simulink model "mmc"  (R2023b)
settings: Solver=VariableStepAuto  StartTime=0.0  StopTime=2  RelTol=1e-3
values from neighbouring files (symbols this model uses):
  ab0_to_cell = inv(cell_to_2ab0)    [init_mmc.m]
  cell_to_2ab0 = kron(abc_to_ab0, abc_to_ab0)    [init_mmc.m]
  grid_to_cell = kron(eye(3), ones(3, 1))    [init_mmc.m]
  J = [0 -1; 1 0]    [SafetyFilterSystemDPC.m]    (also in init_mmc.m)
  machine_to_cell = kron(ones(3, 1), eye(3))    [init_mmc.m]
  volt_to_cell = [      [          1 0 0 0 0 0 ... (first row only)    [init_mmc.m]
undefined symbols (not defined in the file or in its folder): cpu, ctrl, DiscIntNeverNeededParam, fdesignblkfcn, gcbh, grid, load1, machine, mmc, pq_ctrl, sim, soa
libraries: eeDiscretePi x9, spsabctodq0Lib x9, spsThreePhaseSeriesRLCBranchLib x8, dsparch4 x6, spsControlledVoltageSourceLib x6, spsThreePhaseVIMeasurementLib x6, eeGeneralControl x5, spsBreakerLib x3, spsGroundLib x3, library x3, spsThreePhaseBreakerLib x2, spsdq0toabcLib x2
(part 1 of 2)
settings Model: SimulationMode=accelerator  Creator=ma1155716  LastModifiedBy=ma1155716

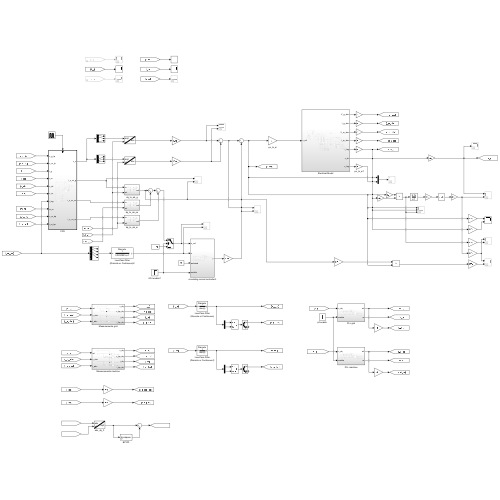
[thumbnail: Simulink's stored preview of the top-level diagram]
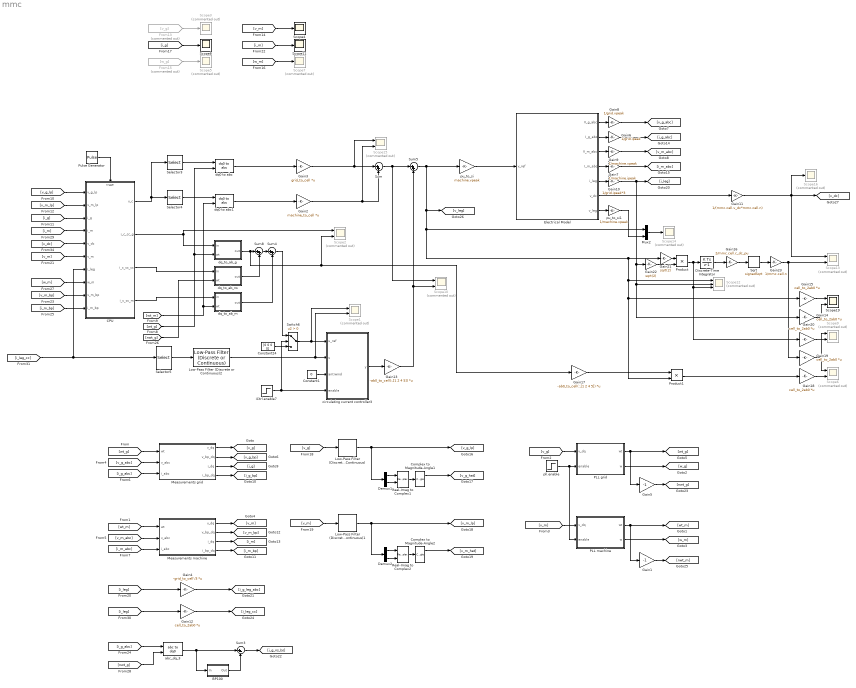
== system mmc ==
  BP100 : Subsystem  DialogController=fdesignblkfcn  InitFcn=fdesignblkfcn(gcbh, {'InitFcn'});  mask(Bandpass Filter){}
      mask help: dsp:DSPFilterDesignBlockDialog:BandpassFdesign_MaskDesc
      settings: CopyFcn=fdesignblkfcn(gcbh, {'CopyFcn'});
      mask Help: helpview(mapfilelocation('dsp'), 'dspbandpassfilter');
      mask Display: disp('Bandpass');
  CPU : Subsystem
  Complex to Magnitude-Angle1 : ComplexToMagnitudeAngle
  Complex to Magnitude-Angle2 : ComplexToMagnitudeAngle
  Constant1 : Constant  Value=0
  Constant24 : Constant  Value=[0 0 0 0]
  Demux1 : Demux  Outputs=2
  Demux2 : Demux  Outputs=2
  Discrete-Time Integrator : DiscreteIntegrator  gainval=1  SampleTime=-1  ICPrevOutput=DiscIntNeverNeededParam  ICPrevScaledInput=DiscIntNeverNeededParam
  Electrical Model : Subsystem
  From13 : From  Commented=on  GotoTag=v_g
  From15 : From  Commented=on  GotoTag=w_g
  Gain1 : Gain  Gain=-1
  Gain10 : Gain  Gain=1/grid.ipeak*3
  Gain11 : Gain  Gain=1/(mmc.cell.v_dc*mmc.cell.n)
  Gain{12,14..15,18..20} (6 alike) : Gain  Gain=cell_to_2ab0  Multiplication=Matrix(K*u)
  Gain13 : Gain  Gain=-ab0_to_cell(:,[1 2 4 5])  Multiplication=Matrix(K*u)
  Gain16 : Gain  Gain=2/mmc.cell.c_dc_pu
  Gain17 : Gain  Gain=-ab0_to_cell(:,[1 2 4 5])  Multiplication=Matrix(K*u)
  Gain2 : Gain  Gain=machine_to_cell  Multiplication=Matrix(K*u)
  Gain21 : Gain  Gain=sqrt(2)
  Gain22 : Gain  Gain=sqrt(2)
  Gain23 : Gain  Gain=1/mmc.cell.n
  Gain3 : Gain  Gain=grid_to_cell  Multiplication=Matrix(K*u)
  Gain4 : Gain  Gain=-grid_to_cell'/3  Multiplication=Matrix(K*u)
  Gain5 : Gain  Gain=-1
  Gain6 : Gain  Gain=1/grid.ipeak
  Gain7 : Gain  Gain=1/machine.ipeak
  Gain8 : Gain  Gain=1/grid.vpeak
  Gain9 : Gain  Gain=1/machine.vpeak
  Low-Pass Filter (Discrete or Continuous) : eeGeneralControl/Low-Pass Filter (Discrete or Continuous)  K=1  T=1/grid.w*10  B=inf  A=-inf  init_option=Specify as parameter  x0=[1 0 0]  Ts=-1
  Low-Pass Filter (Discrete or Continuous)1 : eeGeneralControl/Low-Pass Filter (Discrete or Continuous)  K=1  T=1/machine.w*10  B=inf  A=-inf  init_option=Specify as parameter  x0=[1 0 0]  Ts=-1
  Low-Pass Filter (Discrete or Continuous)2 : eeGeneralControl/Low-Pass Filter (Discrete or Continuous)  K=1  T=1/grid.w  B=inf  A=-inf  init_option=Inherited from block input  x0=0  Ts=-1
  Measurements grid : Subsystem
  Measurements machine : Subsystem
  Mux2 : Mux  Inputs=2
  PLL grid : Subsystem
  PLL machine : Subsystem
  Product : Product
  Product1 : Product
  Pulse Generator : DiscretePulseGenerator  PulseType=Time based  Period=cpu.ts  PulseWidth=50
  Real-Imag to Complex1 : RealImagToComplex
  Real-Imag to Complex2 : RealImagToComplex
  Scope{1..2,6,9..10,13,15} (7 alike) : Scope  Commented=on  NumInputPorts=2
  Scope11 : Scope
  Scope12 : Scope  Commented=on  NumInputPorts=3
  Scope{3,5,7,14,16} (5 alike) : Scope  Commented=on
  Scope19 : Scope  NumInputPorts=2
  Scope4 : Scope
  Scope8 : Scope
  Selector3 : Selector  InputPortWidth=5  IndexOptions=Index vector (dialog)  Indices=[1 2 5]  OutputSizes=1
  Selector4 : Selector  InputPortWidth=5  IndexOptions=Index vector (dialog)  Indices=[3 4 5]  OutputSizes=1
  Selector5 : Selector  InputPortWidth=9  IndexOptions=Index vector (dialog)  Indices=[1 2 4 5]  OutputSizes=1
  Sqrt : Sqrt  Operator=signedSqrt
  Sum{,4..5,8} (4 alike) : Sum  Inputs=|++
  Sum3 : Sum  Inputs=|+-
  Switch6 : Switch  Criteria=u2 > Threshold  SaturateOnIntegerOverflow=off  InputSameDT=off
  abc_dq_3 : spsabctodq0Lib/abc to dq0  Alignment=Aligned with phase A axis
  circulating current controller3 : Subsystem  VariantControl=overcurr_ctrl.sel==1
  dq0 to abc : spsdq0toabcLib/dq0 to abc  Alignment=Aligned with phase A axis
  dq0 to abc1 : spsdq0toabcLib/dq0 to abc  Alignment=Aligned with phase A axis
  dq_to_ab_g : Subsystem
  dq_to_ab_m : Subsystem
  dq_to_ab_ns : Subsystem
  iCtrl.enable7 : Step  Time=ctrl.grid.ictrl.enable
  "pll.enable " : Step  Time=ctrl.grid.pll.enable
  pu_to_si : Gain  Gain=machine.vpeak
  pu_to_si1 : Gain  Gain=1/machine.vpeak
  wires:
  Electrical Model/2(I_g_abc) -> Gain6/1
  Electrical Model/4(I_m_abc) -> Gain7/1
  Pulse Generator/1 -> CPU/Trigger
  "pll.enable "/1 -> PLL machine/2(enable), PLL grid/2(enable)
  PLL grid/1(wt) -> Gain5/1, [wt_g]
  [wt_g] -> Measurements grid/1(wt)
  [wt_m] -> Measurements machine/1(wt)
  PLL grid/2(w) -> [w_g]
  PLL machine/2(w) -> [w_m]
  Measurements grid/1(v_dq) -> [v_g]
  Measurements machine/1(v_dq) -> [v_m]
  [v_m] -> PLL machine/1(v_dq)
  [v_g] -> PLL grid/1(v_dq)
  Measurements grid/2(v_bp_dq) -> [v_g_bp]
  [v_g_abc] -> Measurements grid/2(v_abc)
  [v_m_abc] -> Measurements machine/2(v_abc)
  Electrical Model/1(V_g_abc) -> Gain8/1
  Electrical Model/3(V_m_abc) -> Gain9/1
  [i_g_abc] -> Measurements grid/3(i_abc)
  [i_m_abc] -> Measurements machine/3(i_abc)
  Measurements grid/3(i_dq) -> [i_g]
  Measurements grid/4(i_bp_dq) -> [i_g_bp]
  Measurements machine/2(v_bp_dq) -> [v_m_bp]
  Measurements machine/3(i_dq) -> [i_m]
  Measurements machine/4(i_bp_dq) -> [i_m_bp]
  dq0 to abc/1 -> Gain3/1
  dq0 to abc1/1 -> Gain2/1
  Selector3/1 -> dq0 to abc/1
  Selector4/1 -> dq0 to abc1/1
  CPU/1(v_c) -> Selector4/1, Selector3/1
  Gain3/1 -> Scope15/1, Sum/1
  [v_g_lp] -> CPU/1(v_g_lp)
  [i_g] -> CPU/3(i_g)
  [v_m_lp] -> CPU/2(v_m_lp)
  pu_to_si/1 -> Electrical Model/1(v_ref)
  From13/1 -> Scope3/1
  [v_m] -> Scope4/1
  From15/1 -> Scope5/1
  [w_m] -> Scope7/1
  [i_g] -> Scope8/1
  Low-Pass Filter (Discrete or Continuous)/1 -> [v_g_lp], Demux1/1
  Demux1/1 -> Real-Imag to Complex1/1
  Complex to Magnitude-Angle1/1 -> [v_g_hat]
  Real-Imag to Complex1/1 -> Complex to Magnitude-Angle1/1
  Demux1/2 -> Real-Imag to Complex1/2
  [v_g] -> Low-Pass Filter (Discrete or Continuous)/1
  [v_m] -> Low-Pass Filter (Discrete or Continuous)1/1
  Low-Pass Filter (Discrete or Continuous)1/1 -> [v_m_lp], Demux2/1
  Real-Imag to Complex2/1 -> Complex to Magnitude-Angle2/1
  Demux2/1 -> Real-Imag to Complex2/1
  Demux2/2 -> Real-Imag to Complex2/2
  Complex to Magnitude-Angle2/1 -> [v_m_hat]
  Electrical Model/5(i_leg) -> Gain10/1
  Gain4/1 -> [i_g_leg_abc]
  [i_leg] -> Gain4/1
  Gain6/1 -> [i_g_abc]
  Gain7/1 -> [i_m_abc]
  Gain8/1 -> [v_g_abc]
  Gain9/1 -> [v_m_abc]
  Gain10/1 -> Gain14/1, Scope12/2, Gain22/1, [i_leg]
  [i_g_abc] -> abc_dq_3/1
  [nwt_g] -> abc_dq_3/2
  abc_dq_3/1 -> Sum3/1, BP100/1(In)
  Gain5/1 -> [nwt_g]
  BP100/1(Out) -> Sum3/2
  Sum3/1 -> [i_g_ns_bs]
  [i_m] -> Scope11/1
  [i_m] -> CPU/4(i_m)
  PLL machine/1(wt) -> Gain1/1, [wt_m]
  Gain1/1 -> [nwt_m]
  Product/1 -> Discrete-Time Integrator/1, Scope12/3, Gain20/1
  Gain14/1 -> Scope19/2
  [i_leg] -> Gain12/1
  Gain12/1 -> [i_leg_cc]
  [i_leg_cc] -> Selector5/1, CPU/7(i_leg)
  Discrete-Time Integrator/1 -> Gain16/1
  Gain16/1 -> Sqrt/1
  [v_dc] -> CPU/5(v_dc)
  Gain23/1 -> Scope13/2, Gain19/1
  Gain15/1 -> Scope19/1
  CPU/2(i_c_cc_g) -> Scope2/1, dq_to_ab_g/1(in)
  [nwt_g] -> dq_to_ab_ns/2(wt)
  CPU/3(i_c_cc_cc) -> dq_to_ab_ns/1(in)
  CPU/4(i_c_cc_m) -> dq_to_ab_m/1(in)
  dq_to_ab_g/1(out) -> Scope2/2, Gain17/1, Sum8/1
  Sum8/1 -> Sum4/1
  dq_to_ab_ns/1(out) -> Sum8/2
  dq_to_ab_m/1(out) -> Sum4/2
  [wt_g] -> dq0 to abc/2, dq_to_ab_g/2(wt)
  [wt_m] -> dq0 to abc1/2, dq_to_ab_m/2(wt)
  Constant1/1 -> circulating current controller3/3(antiwind)
  Sum4/1 -> Switch6/1
  Switch6/1 -> circulating current controller3/1(u_ref), Scope1/1
  iCtrl.enable7/1 -> circulating current controller3/4(enable), Switch6/2
  Constant24/1 -> Switch6/3
  Sum/1 -> Sum5/1, Scope10/1
  Gain13/1 -> Sum5/2, Scope10/2
  Product1/1 -> Gain18/1
  Gain17/1 -> Product1/1
  Gain18/1 -> Scope6/2
  Gain19/1 -> Scope9/1, Scope6/1
  Gain20/1 -> Scope9/2
  [v_m] -> CPU/6(v_m)
  circulating current controller3/1(y) -> Gain13/1
  Gain11/1 -> Scope16/1, [v_dc], Scope13/1
  Electrical Model/6(v_dc) -> Gain11/1
  Gain21/1 -> Product/1
  Gain22/1 -> Product/2
  Sqrt/1 -> Gain23/1
  Sum5/1 -> pu_to_si/1, [v_leg], Scope12/1, Product1/2, Gain15/1, Gain21/1, Mux2/1
  Electrical Model/7(v_leg) -> pu_to_si1/1
  pu_to_si1/1 -> Mux2/2
  Mux2/1 -> Scope14/1
  Gain2/1 -> Scope15/2, Sum/2
  Selector5/1 -> Low-Pass Filter (Discrete or Continuous)2/1
  Low-Pass Filter (Discrete or Continuous)2/1 -> circulating current controller3/2(u), Scope1/2
  [i_m_bp] -> CPU/10(i_m_bp)
  [v_m_bp] -> CPU/9(v_m_bp)
  [w_m] -> CPU/8(w_m)

== system mmc/BP100 ==
  In : Inport
  Generated Filter Block : dsparch4/Biquad Filter  Tag=BlockMethodSubSystem  FilterSource=Dialog parameters  CoeffSource=Specify via dialog  FilterObject=BQF  IIRFiltStruct=Direct form II  BiQuadCoeffs=[2 0 -2 1 -1.99993786796251327 0.999938262487757412]  ScaleValues=[1.99433834389553329e-07;77.3909708347894423]  IC=0  ICnum=0  ICden=0  a0Flag=Warning  optimizeScaleValues=off  ScaleValueMode=Specify via input port (g)  roundingMode=Floor  overflowMode=off  scaleValueFracLength=14  denProdOutputFracLength=30  denAccumFracLength=30  secondMemoryFracLength=15
  Out : Outport  VectorParamsAs1DForOutWhenUnconnected=off
  wires:
  In/1 -> Generated Filter Block/1
  Generated Filter Block/1 -> Out/1

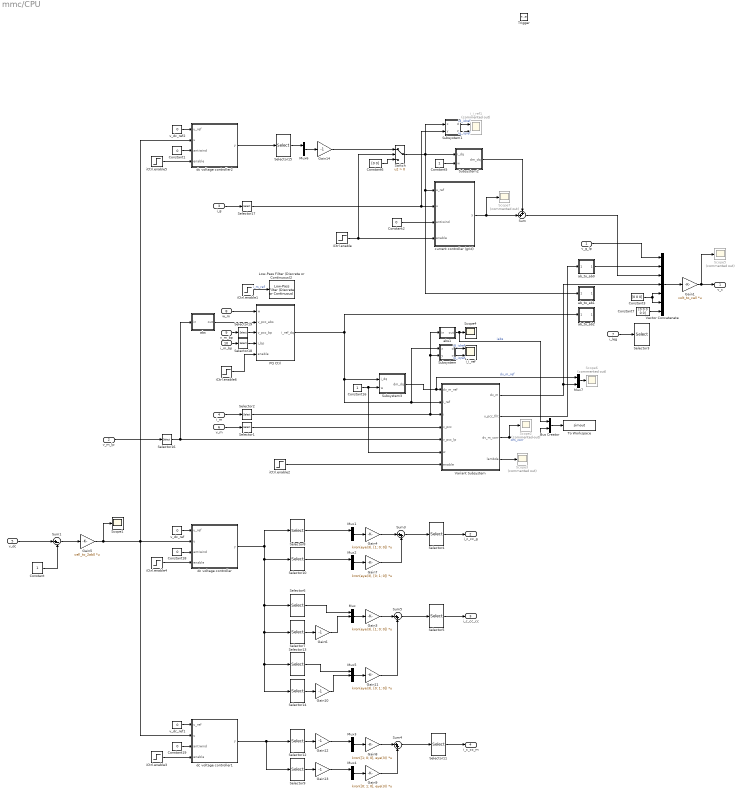
== system mmc/CPU ==
  v_g_lp : Inport
  v_m_lp : Inport  Port=2
  i_g : Inport  Port=3
  i_m : Inport  Port=4
  v_dc : Inport  Port=5
  v_m : Inport  Port=6
  i_leg : Inport  Port=7
  w_m : Inport  Port=8
  v_m_bp : Inport  Port=9
  i_m_bp : Inport  Port=10
  Trigger : TriggerPort  VariantControl=(inherit)
  Bus Creator : BusCreator  Inputs=2
  Constant : Constant
  Constant{1..2,18..19} (4 alike) : Constant  Value=0
  Constant16 : Constant
  Constant3 : Constant  Value=[0 0 0]
  Constant5 : Constant
  Constant6 : Constant  Value=[0 0]
  Constant7 : Constant  Value=[0 0 0 0 0]
  Gain1 : Gain  Gain=volt_to_cell  Multiplication=Matrix(K*u)
  Gain{6,10,12..14} (5 alike) : Gain  Gain=-1
  Gain11 : Gain  Gain=kron(eye(3), [0; 1; 0])  Multiplication=Matrix(K*u)
  Gain3 : Gain  Gain=kron(eye(3), [1; 0; 0])  Multiplication=Matrix(K*u)
  Gain4 : Gain  Gain=kron(eye(3), [1; 0; 0])  Multiplication=Matrix(K*u)
  Gain5 : Gain  Gain=cell_to_2ab0  Multiplication=Matrix(K*u)
  Gain7 : Gain  Gain=kron(eye(3), [0; 1; 0])  Multiplication=Matrix(K*u)
  Gain8 : Gain  Gain=kron([1; 0; 0], eye(3))  Multiplication=Matrix(K*u)
  Gain9 : Gain  Gain=kron([0; 1; 0], eye(3))  Multiplication=Matrix(K*u)
  Low-Pass Filter (Discrete or Continuous)2 : eeGeneralControl/Low-Pass Filter (Discrete or Continuous)  K=1  T=0.1  B=inf  A=-inf  init_option=Inherited from block input  x0=0  Ts=-1
  Mux{,1..5} (6 alike) : Mux  Inputs=3
  Mux6 : Mux  Inputs=2
  Mux7 : Mux  Inputs=2
  PQ Ctrl : Subsystem
  Scope1 : Scope
  Scope{2..3,5..7} (5 alike) : Scope  Commented=on
  Scope4 : Scope
  Selector{1..2,16..19} (6 alike) : Selector  InputPortWidth=3  IndexOptions=Index vector (dialog)  Indices=[1 2]  OutputSizes=1
  Selector10 : Selector  InputPortWidth=9  IndexOptions=Index vector (dialog)  Indices=[8]  OutputSizes=1
  Selector11 : Selector  InputPortWidth=9  IndexOptions=Index vector (dialog)  Indices=[1 2 4 5]  OutputSizes=1
  Selector12 : Selector  InputPortWidth=9  IndexOptions=Index vector (dialog)  Indices=[3]  OutputSizes=1
  Selector13 : Selector  InputPortWidth=9  IndexOptions=Index vector (dialog)  Indices=[2]  OutputSizes=1
  Selector14 : Selector  InputPortWidth=9  IndexOptions=Index vector (dialog)  Indices=[5]  OutputSizes=1
  Selector15 : Selector  InputPortWidth=9  IndexOptions=Index vector (dialog)  Indices=[9]  OutputSizes=1
  Selector3 : Selector  InputPortWidth=9  IndexOptions=Index vector (dialog)  Indices=[3 6 7 8 9]  OutputSizes=1
  Selector4 : Selector  InputPortWidth=9  IndexOptions=Index vector (dialog)  Indices=[1 2 4 5]  OutputSizes=1
  Selector5 : Selector  InputPortWidth=9  IndexOptions=Index vector (dialog)  Indices=[1 2 4 5]  OutputSizes=1
  Selector6 : Selector  InputPortWidth=9  IndexOptions=Index vector (dialog)  Indices=[1]  OutputSizes=1
  Selector7 : Selector  InputPortWidth=9  IndexOptions=Index vector (dialog)  Indices=[4]  OutputSizes=1
  Selector8 : Selector  InputPortWidth=9  IndexOptions=Index vector (dialog)  Indices=[7]  OutputSizes=1
  Selector9 : Selector  InputPortWidth=9  IndexOptions=Index vector (dialog)  Indices=[6]  OutputSizes=1
  Subsystem : Subsystem
  Subsystem1 : Subsystem
  Subsystem2 : Subsystem
  Subsystem3 : Subsystem
  Sum : Sum  Inputs=++|
  Sum1 : Sum  Inputs=|+-
  Sum3 : Sum  Inputs=|++
  Sum4 : Sum  Inputs=|++
  Sum5 : Sum  Inputs=|++
  Switch : Switch  Criteria=u2 > Threshold  SaturateOnIntegerOverflow=off  InputSameDT=off
  To Workspace : ToWorkspace  VariableName=simout  SaveFormat=Timeseries  SampleTime=-1
  Variant Subsystem : Subsystem  Variant=on
  Vector Concatenate : Concatenate  NumInputs=7
  ab_to_ab0 : Subsystem
  ab_to_ab1 : Subsystem
  ab_to_ab2 : Subsystem
  abs : Subsystem
  abs1 : Subsystem
  current controller (grid) : Subsystem  VariantControl=overcurr_ctrl.sel==1
  dc voltage controller : Subsystem  VariantControl=overcurr_ctrl.sel==1
  dc voltage controller1 : Subsystem  VariantControl=overcurr_ctrl.sel==1
  dc voltage controller2 : Subsystem  VariantControl=overcurr_ctrl.sel==1
  iCtrl.enable : Step  Time=ctrl.grid.ictrl.enable
  iCtrl.enable1 : Step  Time=ctrl.machine.ictrl.ref_enable  Before=[0 0]  After=[1.18 0]
  iCtrl.enable2 : Step  Time=ctrl.machine.ictrl.enable
  iCtrl.enable3 : Step  Time=ctrl.grid.ictrl.enable
  iCtrl.enable4 : Step  Time=ctrl.grid.ictrl.enable
  iCtrl.enable5 : Step  Time=grid.breaker_close
  iCtrl.enable6 : Step  Time=ctrl.machine.ictrl.enable
  i_i_ref : Scope  NumInputPorts=2
  i_i_ref1 : Scope  Commented=on  NumInputPorts=2
  v_dc_ref : Constant  Value=0
  v_dc_ref1 : Constant  Value=0
  v_dc_ref2 : Constant  Value=0
  v_c : Outport
  i_c_cc_g : Outport  Port=2
  i_c_cc_cc : Outport  Port=3
  i_c_cc_m : Outport  Port=4
  wires:
  Switch/1 -> Subsystem1/1(x), Subsystem2/1(i_dq), ab_to_ab1/1(In1), current controller (grid)/1(u_ref)
  i_g/1 -> Selector17/1
  Constant2/1 -> current controller (grid)/3(antiwind)
  Vector Concatenate/1 -> Gain1/1
  Gain1/1 -> Scope5/1, v_c/1
  Selector17/1 -> Subsystem1/2(y), current controller (grid)/2(u)
  v_g_lp/1 -> Vector Concatenate/1
  v_m_lp/1 -> Selector16/1
  Subsystem2/1(dm_dq) -> Sum/1
  Constant5/1 -> Subsystem2/2(w)
  Constant6/1 -> Switch/3
  Sum/1 -> Vector Concatenate/3
  current controller (grid)/1(y) -> Scope7/1, Sum/2
  iCtrl.enable/1 -> Switch/2, current controller (grid)/4(enable)
  iCtrl.enable1/1 -> Low-Pass Filter (Discrete or Continuous)2/1  "i_m_ref"
  Constant16/1 -> Subsystem3/2(w), Variant Subsystem/6(w)
  i_m/1 -> Selector2/1
  iCtrl.enable2/1 -> Variant Subsystem/7(enable)
  Selector4/1 -> i_c_cc_g/1
  Gain4/1 -> Sum3/1
  v_dc_ref/1 -> dc voltage controller/1(u_ref)
  iCtrl.enable4/1 -> dc voltage controller/4(enable)
  Constant18/1 -> dc voltage controller/3(antiwind)
  Selector6/1 -> Mux/1
  Selector7/1 -> Gain6/1
  Gain6/1 -> Mux/2
  Selector8/1 -> Mux1/1
  Mux/1 -> Gain3/1
  Mux1/1 -> Gain4/1
  Selector5/1 -> i_c_cc_cc/1
  Selector10/1 -> Mux2/1
  Mux2/1 -> Gain7/1
  Sum3/1 -> Selector4/1
  Selector12/1 -> Gain12/1
  Mux3/1 -> Gain8/1
  Gain8/1 -> Sum4/1
  Selector9/1 -> Gain13/1
  Selector11/1 -> i_c_cc_m/1
  Mux4/1 -> Gain9/1
  Sum4/1 -> Selector11/1
  Gain9/1 -> Sum4/2
  dc voltage controller/1(y) -> Selector10/1, Selector13/1, Selector14/1, Selector7/1, Selector6/1, Selector8/1
  Selector14/1 -> Gain10/1
  Selector13/1 -> Mux5/1
  Gain10/1 -> Mux5/2
  Mux5/1 -> Gain11/1
  Sum5/1 -> Selector5/1
  Gain12/1 -> Mux3/1
  Gain13/1 -> Mux4/1
  Gain3/1 -> Sum5/1
  Selector15/1 -> Mux6/1
  Gain14/1 -> Switch/1
  Gain7/1 -> Sum3/2
  Gain11/1 -> Sum5/2
  v_dc_ref1/1 -> dc voltage controller1/1(u_ref)
  Constant19/1 -> dc voltage controller1/3(antiwind)
  iCtrl.enable3/1 -> dc voltage controller1/4(enable)
  Sum1/1 -> Gain5/1
  dc voltage controller1/1(y) -> Selector9/1, Selector12/1
  Mux6/1 -> Gain14/1
  Gain5/1 -> dc voltage controller2/2(u), dc voltage controller1/2(u), dc voltage controller/2(u), Scope1/1
  v_dc_ref2/1 -> dc voltage controller2/1(u_ref)
  Constant1/1 -> dc voltage controller2/3(antiwind)
  iCtrl.enable5/1 -> dc voltage controller2/4(enable)
  dc voltage controller2/1(y) -> Selector15/1
  Subsystem3/1(dm_dq) -> Mux7/1, Variant Subsystem/1(dv_m_ref)  "dv_m_ref"
  Selector2/1 -> abs1/1(in), Subsystem/2(y), Variant Subsystem/3(i)
  Variant Subsystem/1(dv_m) -> Vector Concatenate/4, Mux7/2
  v_m/1 -> Selector1/1
  Selector1/1 -> Variant Subsystem/4(v_pcc)
  Variant Subsystem/4(lambda) -> Scope3/1
  Variant Subsystem/3(dv_m_corr) -> Bus Creator/2, Scope2/1  "dm_corr"
  Selector16/1 -> Variant Subsystem/5(v_pcc_lp), abs/1(in)
  v_dc/1 -> Sum1/1
  Constant/1 -> Sum1/2
  i_leg/1 -> Selector3/1
  Variant Subsystem/2(v_pcc_filt) -> ab_to_ab0/1(In1)
  ab_to_ab0/1(Out1) -> Vector Concatenate/2
  w_m/1 -> PQ Ctrl/1(w)
  abs/1(out) -> PQ Ctrl/2(v_pcc_abs)
  v_m_bp/1 -> Selector19/1
  i_m_bp/1 -> Selector18/1
  Selector18/1 -> PQ Ctrl/4(i_bp)
  Selector19/1 -> PQ Ctrl/3(v_pcc_bp)
  iCtrl.enable6/1 -> PQ Ctrl/5(enable)
  PQ Ctrl/1(i_ref_dq) -> ab_to_ab2/1(i_ref_dq), Subsystem/1(x), Variant Subsystem/2(i_ref), Subsystem3/1(i_dq)
  abs1/1(out) -> Bus Creator/1, Scope4/1  "iabs"
  Mux7/1 -> Scope6/1
  Subsystem/1(d) -> i_i_ref/1  "id_idref"
  Subsystem/2(q) -> i_i_ref/2  "iq_iqref"
  Constant7/1 -> Vector Concatenate/7
  Constant3/1 -> Vector Concatenate/6, Vector Concatenate/5
  Subsystem1/2(q) -> i_i_ref1/2  "iq_iqref"
  Subsystem1/1(d) -> i_i_ref1/1  "id_idref"
  Bus Creator/1 -> To Workspace/1

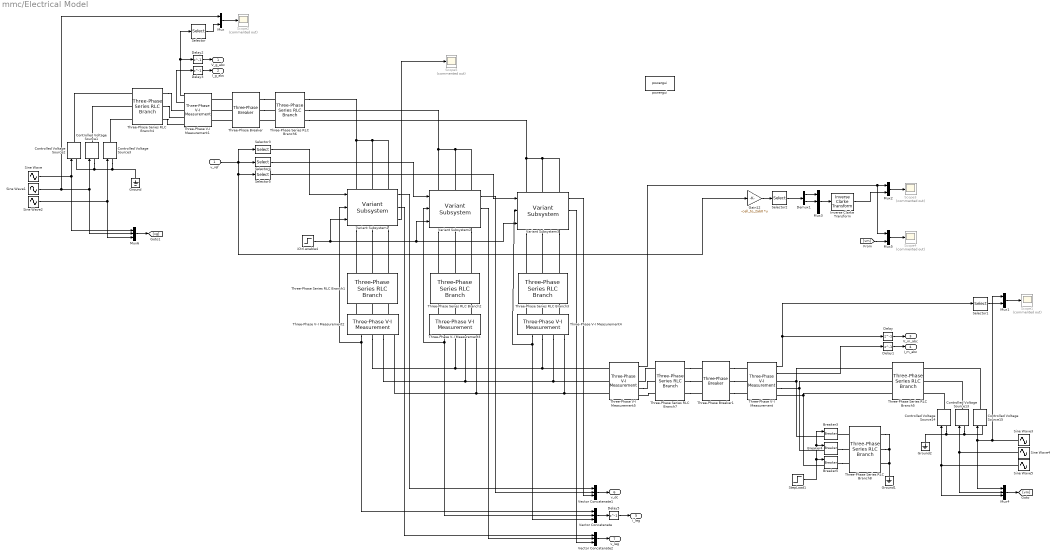
== system mmc/Electrical Model ==
  v_ref : Inport
  Breaker3 : spsBreakerLib/Breaker  InitialState=0  SwitchingTimes="[1/60  5/60]"  External=on  BreakerResistance=0.01  SnubberResistance=1e6  SnubberCapacitance=inf  Measurements=None  MoreParameters=on  NoBreakLoop=off
  Breaker4 : spsBreakerLib/Breaker  InitialState=0  SwitchingTimes="[1/60  5/60]"  External=on  BreakerResistance=0.01  SnubberResistance=1e6  SnubberCapacitance=inf  Measurements=None  MoreParameters=on  NoBreakLoop=off
  Breaker5 : spsBreakerLib/Breaker  InitialState=0  SwitchingTimes="[1/60  5/60]"  External=on  BreakerResistance=0.01  SnubberResistance=1e6  SnubberCapacitance=inf  Measurements=None  MoreParameters=on  NoBreakLoop=off
  Controlled Voltage Source{1..3,13..15} (6 alike) : spsControlledVoltageSourceLib/Controlled Voltage Source  Initialize=on  Source_Type=AC  Amplitude=0  Phase=0  Frequency=0  Measurements=None
  Delay{,1..3,5} (5 alike) : Delay  DelayLength=1  InitialCondition=0  SampleTime=sim.ts
  Demux1 : Demux  Outputs=2
  Gain12 : Gain  Gain=-cell_to_2ab0  Multiplication=Matrix(K*u)
  Ground : spsGroundLib/Ground  LConnTagsString=a
  Ground1 : spsGroundLib/Ground  LConnTagsString=a
  Ground2 : spsGroundLib/Ground  LConnTagsString=a
  Inverse Clarke Transform : eeTransforms/Inverse Clarke Transform  PowerInvariant=off
      settings: LibrarySourceBlock=|
      | ee_sl_lib/Mathematical
      | Transforms/Inverse
      | Clarke Transform
  Mux{,1..2,5} (4 alike) : Mux  Inputs=2
  Mux3 : Mux  Inputs=3
  Mux4 : Mux  Inputs=3
  Mux6 : Mux  Inputs=3
  Scope{1..5} (5 alike) : Scope  Commented=on
  Selector : Selector  InputPortWidth=3  IndexOptions=Index vector (dialog)  Indices=[2]  OutputSizes=1
  Selector1 : Selector  InputPortWidth=3  IndexOptions=Index vector (dialog)  Indices=[1]  OutputSizes=1
  Selector2 : Selector  InputPortWidth=9  IndexOptions=Index vector (dialog)  Indices=[7 8]  OutputSizes=1
  Selector3 : Selector  InputPortWidth=9  IndexOptions=Index vector (dialog)  Indices=[1 2 3]  OutputSizes=1
  Selector4 : Selector  InputPortWidth=9  IndexOptions=Index vector (dialog)  Indices=[4 5 6]  OutputSizes=1
  Selector5 : Selector  InputPortWidth=9  IndexOptions=Index vector (dialog)  Indices=[7 8 9]  OutputSizes=1
  Sine Wave : Sin  Amplitude=grid.vpeak  Frequency=grid.w  Phase=pi/2  SampleTime=0
  Sine Wave1 : Sin  Amplitude=grid.vpeak  Frequency=grid.w  Phase=pi/2-2*pi/3  SampleTime=0
  Sine Wave2 : Sin  Amplitude=grid.vpeak  Frequency=grid.w  Phase=pi/2+2*pi/3  SampleTime=0
  Sine Wave3 : Sin  Amplitude=machine.vpeak  Frequency=machine.w_set  Phase=pi/2  SampleTime=0
  Sine Wave4 : Sin  Amplitude=machine.vpeak  Frequency=machine.w_set  Phase=pi/2-2*pi/3  SampleTime=0
  Sine Wave5 : Sin  Amplitude=machine.vpeak  Frequency=machine.w_set  Phase=pi/2+2*pi/3  SampleTime=0
  StepLoad1 : Step  Time=load1.stepTime  SampleTime=0
  Three-Phase Series RLC Branch1 : spsThreePhaseSeriesRLCBranchLib/Three-Phase Series RLC Branch  LConnTagsString=A|B|C  RConnTagsString=A|B|C  BranchType=RL  Resistance=mmc.r_leg_si  Inductance=mmc.l_leg_si  Capacitance=1e-6  Measurements=None
  Three-Phase Series RLC Branch2 : spsThreePhaseSeriesRLCBranchLib/Three-Phase Series RLC Branch  LConnTagsString=A|B|C  RConnTagsString=A|B|C  BranchType=RL  Resistance=mmc.r_leg_si  Inductance=mmc.l_leg_si  Capacitance=1e-6  Measurements=None
  Three-Phase Series RLC Branch3 : spsThreePhaseSeriesRLCBranchLib/Three-Phase Series RLC Branch  LConnTagsString=A|B|C  RConnTagsString=A|B|C  BranchType=RL  Resistance=mmc.r_leg_si  Inductance=mmc.l_leg_si  Capacitance=1e-6  Measurements=None
  Three-Phase Series RLC Branch4 : spsThreePhaseSeriesRLCBranchLib/Three-Phase Series RLC Branch  LConnTagsString=A|B|C  RConnTagsString=A|B|C  BranchType=RL  Resistance=grid.tr.r_si*0.1  Inductance=grid.tr.l_si*0.1  Capacitance=1e-6  Measurements=None
  Three-Phase Series RLC Branch5 : spsThreePhaseSeriesRLCBranchLib/Three-Phase Series RLC Branch  LConnTagsString=A|B|C  RConnTagsString=A|B|C  BranchType=RL  Resistance=machine.tr.r_si*0.1  Inductance=machine.tr.l_si*0.1  Capacitance=1e-6  Measurements=None
  Three-Phase Series RLC Branch6 : spsThreePhaseSeriesRLCBranchLib/Three-Phase Series RLC Branch  LConnTagsString=A|B|C  RConnTagsString=A|B|C  BranchType=RL  Resistance=grid.tr.r_si  Inductance=grid.tr.l_si  Capacitance=1e-6  Measurements=None
  Three-Phase Series RLC Branch7 : spsThreePhaseSeriesRLCBranchLib/Three-Phase Series RLC Branch  LConnTagsString=A|B|C  RConnTagsString=A|B|C  BranchType=RL  Resistance=machine.tr.r_si  Inductance=machine.tr.l_si  Capacitance=1e-6  Measurements=None
  Three-Phase Series RLC Branch8 : spsThreePhaseSeriesRLCBranchLib/Three-Phase Series RLC Branch  LConnTagsString=A|B|C  RConnTagsString=A|B|C  BranchType=RL  Resistance=machine.tr.r_si*0.1  Inductance=machine.tr.l_si*0.1  Capacitance=1e-6  Measurements=None
  Three-Phase V-I Measurement{,1..5} (6 alike) : spsThreePhaseVIMeasurementLib/Three-Phase V-I Measurement  VoltageMeasurement=phase-to-ground  SetLabelV=off  LabelV=Vabc  Vpu=off  VpuLL=off  CurrentMeasurement=yes  SetLabelI=off  LabelI=Iabc  Ipu=off  Pbase=100e6  Vbase=500e3  OutputType=Complex  PhasorSimulation=off  PSBequivalent=0
  Three-Phase Breaker : spsThreePhaseBreakerLib/Three-Phase Breaker  InitialState=open  SwitchA=on  SwitchB=on  SwitchC=on  SwitchTimes=[grid.breaker_close]  External=off  BreakerResistance=0.01  SnubberResistance=1e6  SnubberCapacitance=inf  Measurements=None
  Three-Phase Breaker1 : spsThreePhaseBreakerLib/Three-Phase Breaker  InitialState=open  SwitchA=on  SwitchB=on  SwitchC=on  SwitchTimes=[machine.breaker_close]  External=off  BreakerResistance=0.01  SnubberResistance=1e6  SnubberCapacitance=inf  Measurements=None
  Variant Subsystem1 : library/Variant Subsystem  SystemSampleTime=-1  VariantActivationTime=update diagram  AllowFlexibleInterface=on  Latency=0  AutoFrameSizeCalculation=off
      settings: PortSchema="{\"entries\":[{\"content\":{\"sides\":[{\"content\":{\"connectorIds\":[\"In1\",\"In2\",\"In3\"]},\"type\":\"ConnectorPlacement.EquallySpacedRectSide\",\"uuid\":\"07cc1b48-4eec-48c8-b7e1-ba85327af049\"},{\"content\":{\"connectorIds\":[\"Out1\",\"Out2\",\"Out3\"],\"side\":\"RIGHT\"},\"type\":\"ConnectorPlacement.EquallySpacedRectSide\",\"uuid\":\"e630ccd2-bced-4562-b965-5ba67d1cb520\"},{\"content\":{\"connectorIds\":[\"LConn1\",\"LConn2\",\"LConn3\"],\"side\":\"TOP\"},\"type\":\"ConnectorPlacement.EquallySpacedRectSide\",\"uuid\":\"f7ee33a5-0b9e-482c-ae72-b6ca50f6d328\"},{\"content\":{\"connectorIds\":[\"RConn1\",\"RConn2\",\"RConn3\"],\"side\":\"BOTTOM\"},\"type\":\"ConnectorPlacement.EquallySpacedRectSide\",\"uuid\":\"76c11136-f7c0-446b-9aed-353e2cf8a045\"}]},\"type\":\"ConnectorPlacement.EquallySpacedConnector\",\"uuid\":\"ad2af07b-650a-4f66-848d-c3c749fafa1e\"}],\"packageUris\":[\"http://schema.mathworks.com/mf0/Connector/R2020b\"],\"version\":\"1.0\"}"
  Variant Subsystem2 : library/Variant Subsystem  SystemSampleTime=-1  VariantActivationTime=update diagram  AllowFlexibleInterface=on  Latency=0  AutoFrameSizeCalculation=off
      settings: PortSchema="{\"entries\":[{\"content\":{\"sides\":[{\"content\":{\"connectorIds\":[\"In1\",\"In2\",\"In3\"]},\"type\":\"ConnectorPlacement.EquallySpacedRectSide\",\"uuid\":\"07cc1b48-4eec-48c8-b7e1-ba85327af049\"},{\"content\":{\"connectorIds\":[\"Out1\",\"Out2\",\"Out3\"],\"side\":\"RIGHT\"},\"type\":\"ConnectorPlacement.EquallySpacedRectSide\",\"uuid\":\"e630ccd2-bced-4562-b965-5ba67d1cb520\"},{\"content\":{\"connectorIds\":[\"LConn1\",\"LConn2\",\"LConn3\"],\"side\":\"TOP\"},\"type\":\"ConnectorPlacement.EquallySpacedRectSide\",\"uuid\":\"f7ee33a5-0b9e-482c-ae72-b6ca50f6d328\"},{\"content\":{\"connectorIds\":[\"RConn1\",\"RConn2\",\"RConn3\"],\"side\":\"BOTTOM\"},\"type\":\"ConnectorPlacement.EquallySpacedRectSide\",\"uuid\":\"76c11136-f7c0-446b-9aed-353e2cf8a045\"}]},\"type\":\"ConnectorPlacement.EquallySpacedConnector\",\"uuid\":\"ad2af07b-650a-4f66-848d-c3c749fafa1e\"}],\"packageUris\":[\"http://schema.mathworks.com/mf0/Connector/R2020b\"],\"version\":\"1.0\"}"
  Variant Subsystem3 : library/Variant Subsystem  SystemSampleTime=-1  VariantActivationTime=update diagram  AllowFlexibleInterface=on  Latency=0  AutoFrameSizeCalculation=off
      settings: PortSchema="{\"entries\":[{\"content\":{\"sides\":[{\"content\":{\"connectorIds\":[\"In1\",\"In2\",\"In3\"]},\"type\":\"ConnectorPlacement.EquallySpacedRectSide\",\"uuid\":\"07cc1b48-4eec-48c8-b7e1-ba85327af049\"},{\"content\":{\"connectorIds\":[\"Out1\",\"Out2\",\"Out3\"],\"side\":\"RIGHT\"},\"type\":\"ConnectorPlacement.EquallySpacedRectSide\",\"uuid\":\"e630ccd2-bced-4562-b965-5ba67d1cb520\"},{\"content\":{\"connectorIds\":[\"LConn1\",\"LConn2\",\"LConn3\"],\"side\":\"TOP\"},\"type\":\"ConnectorPlacement.EquallySpacedRectSide\",\"uuid\":\"f7ee33a5-0b9e-482c-ae72-b6ca50f6d328\"},{\"content\":{\"connectorIds\":[\"RConn1\",\"RConn2\",\"RConn3\"],\"side\":\"BOTTOM\"},\"type\":\"ConnectorPlacement.EquallySpacedRectSide\",\"uuid\":\"76c11136-f7c0-446b-9aed-353e2cf8a045\"}]},\"type\":\"ConnectorPlacement.EquallySpacedConnector\",\"uuid\":\"ad2af07b-650a-4f66-848d-c3c749fafa1e\"}],\"packageUris\":[\"http://schema.mathworks.com/mf0/Connector/R2020b\"],\"version\":\"1.0\"}"
  Vector Concatenate : Concatenate  NumInputs=3
  Vector Concatenate1 : Concatenate  NumInputs=3
  Vector Concatenate2 : Concatenate  NumInputs=3
  iCtrl.enable4 : Step  Time=ctrl.grid.ictrl.enable
  powergui : sps_lib/powergui  Priority=1  SimulationMode=Discrete  SampleTime=sim.ts  frequency=60  Iterations=50  frequencyindice=0  Pbase=100e6  ErrMax=1e-4  UnitsV=kV  UnitsW=MW  buscounter=0  FunctionMessages=off  echomessages=off  EnableUseOfTLC=off  CurrentSourceSwitches=off  DisableSnubberDevices=off  DisableRonSwitches=off  DisableVfSwitches=off  DisplayEquations=off  AutomaticDiscreteSolvers=off  SolverType=Tustin/Backward Euler (TBE)  Interpol=off  ExternalGateDelay=off  methode=off  Ts=100  x0status=blocks  SPID=on  SwTol=0  HookPort=off  NonlinearTolerance=1e-4  nMaxIteration=100  ContinueOnMaxIteration=off  RestoreLinks=warning  ResistiveCurrentMeasurement=off  Frange=[0:2:500]  Ylog=off  Xlog=on  ShowGrid=off  save=off  variable=ZData  structure=0  ZoomFFT=off  StartTime=0.0  cycles=1  DisplayStyle=1  fundamental=60  FreqAxis=off  MaxFrequency=1000  frequencyindicesteady=1  RmsSteady=1  display=off
  V_g_abc : Outport
  I_g_abc : Outport  Port=2
  V_m_abc : Outport  Port=3
  I_m_abc : Outport  Port=4
  i_leg : Outport  Port=5
  v_dc : Outport  Port=6
  v_leg : Outport  Port=7
  wires:
  Three-Phase V-I Measurement1/1 -> Delay2/1, Selector/1
  Three-Phase V-I Measurement/2 -> Delay1/1
  Sine Wave5/1 -> Mux4/3, Controlled Voltage Source14/1
  Sine Wave1/1 -> Mux/1, Controlled Voltage Source1/1, Mux6/2
  Sine Wave/1 -> Controlled Voltage Source2/1, Mux6/1
  Sine Wave3/1 -> Mux4/1, Controlled Voltage Source15/1, Mux1/1
  Sine Wave2/1 -> Mux6/3, Controlled Voltage Source3/1
  Sine Wave4/1 -> Mux4/2, Controlled Voltage Source13/1
  Three-Phase V-I Measurement/1 -> Selector1/1, Delay/1
  Three-Phase V-I Measurement1/2 -> Delay3/1
  Selector/1 -> Mux/2
  Mux/1 -> Scope2/1
  Selector1/1 -> Mux1/2
  Mux1/1 -> Scope1/1
  Three-Phase V-I Measurement2/2 -> Variant Subsystem1/2, Vector Concatenate/1
  Three-Phase V-I Measurement3/2 -> Variant Subsystem2/2, Vector Concatenate/2
  Three-Phase V-I Measurement4/2 -> Variant Subsystem3/2, Vector Concatenate/3
  Delay/1 -> V_m_abc/1
  Delay1/1 -> I_m_abc/1
  Delay2/1 -> V_g_abc/1
  Delay3/1 -> I_g_abc/1
  Delay5/1 -> i_leg/1
  StepLoad1/1 -> Breaker3/1, Breaker4/1, Breaker5/1
  Vector Concatenate/1 -> Delay5/1
  Variant Subsystem1/1 -> Vector Concatenate1/1
  Variant Subsystem2/1 -> Vector Concatenate1/2
  Variant Subsystem3/1 -> Vector Concatenate1/3
  Vector Concatenate1/1 -> v_dc/1
  Vector Concatenate2/1 -> v_leg/1
  Variant Subsystem1/2 -> Vector Concatenate2/1
  Variant Subsystem2/2 -> Vector Concatenate2/2
  Variant Subsystem3/2 -> Vector Concatenate2/3
  Three-Phase V-I Measurement5/1 -> Mux5/1, Mux2/1
  Mux2/1 -> Scope3/1
  v_ref/1 -> Gain12/1, Selector5/1, Selector4/1, Selector3/1
  Gain12/1 -> Selector2/1
  Selector2/1 -> Demux1/1
  Demux1/1 -> Mux3/1
  Demux1/2 -> Mux3/2
  Mux3/1 -> Inverse Clarke Transform/1
  Inverse Clarke Transform/1 -> Mux2/2
  iCtrl.enable4/1 -> Variant Subsystem1/3, Variant Subsystem3/3, Variant Subsystem2/3
  Selector3/1 -> Variant Subsystem1/1
  Selector4/1 -> Variant Subsystem2/1
  Selector5/1 -> Variant Subsystem3/1
  Mux4/1 -> [vm]
  [vm] -> Mux5/2
  Mux5/1 -> Scope4/1
  Mux6/1 -> [vg]
  Variant Subsystem1/3 -> Scope5/1
  connections:
  Three-Phase Series RLC Branch6/RConn1 -- Variant Subsystem1/LConn1 -- Variant Subsystem1/LConn2 -- Variant Subsystem1/LConn3
  Ground/LConn1 -- Controlled Voltage Source2/LConn1 -- Controlled Voltage Source1/LConn1 -- Controlled Voltage Source3/LConn1
  Ground2/LConn1 -- Controlled Voltage Source14/LConn1 -- Controlled Voltage Source15/LConn1 -- Controlled Voltage Source13/LConn1
  Controlled Voltage Source15/RConn1 -- Three-Phase Series RLC Branch5/RConn1
  Three-Phase Series RLC Branch6/RConn2 -- Variant Subsystem2/LConn1 -- Variant Subsystem2/LConn3 -- Variant Subsystem2/LConn2
  Three-Phase V-I Measurement2/RConn1 -- Three-Phase V-I Measurement3/RConn1 -- Three-Phase V-I Measurement5/LConn1 -- Three-Phase V-I Measurement4/RConn1
  Controlled Voltage Source1/RConn1 -- Three-Phase Series RLC Branch4/LConn2
  Three-Phase Series RLC Branch4/RConn1 -- Three-Phase V-I Measurement1/RConn1
  Three-Phase Series RLC Branch5/LConn1 -- Breaker3/LConn1 -- Three-Phase V-I Measurement/RConn1
  Three-Phase Series RLC Branch6/RConn3 -- Variant Subsystem3/LConn1 -- Variant Subsystem3/LConn2 -- Variant Subsystem3/LConn3
  Three-Phase Series RLC Branch4/RConn3 -- Three-Phase V-I Measurement1/RConn3
  Three-Phase Series RLC Branch5/LConn3 -- Breaker5/LConn1 -- Three-Phase V-I Measurement/RConn3
  Three-Phase V-I Measurement2/RConn2 -- Three-Phase V-I Measurement3/RConn2 -- Three-Phase V-I Measurement5/LConn2 -- Three-Phase V-I Measurement4/RConn2
  Controlled Voltage Source3/RConn1 -- Three-Phase Series RLC Branch4/LConn3
  Three-Phase Series RLC Branch4/RConn2 -- Three-Phase V-I Measurement1/RConn2
  Controlled Voltage Source2/RConn1 -- Three-Phase Series RLC Branch4/LConn1
  Three-Phase V-I Measurement2/RConn3 -- Three-Phase V-I Measurement5/LConn3 -- Three-Phase V-I Measurement4/RConn3 -- Three-Phase V-I Measurement3/RConn3
  Controlled Voltage Source14/RConn1 -- Three-Phase Series RLC Branch5/RConn3
  Three-Phase V-I Measurement/RConn2 -- Breaker4/LConn1 -- Three-Phase Series RLC Branch5/LConn2
  Controlled Voltage Source13/RConn1 -- Three-Phase Series RLC Branch5/RConn2
  Three-Phase V-I Measurement2/LConn1 -- Three-Phase Series RLC Branch1/RConn1
  Three-Phase V-I Measurement2/LConn2 -- Three-Phase Series RLC Branch1/RConn2
  Three-Phase V-I Measurement2/LConn3 -- Three-Phase Series RLC Branch1/RConn3
  Three-Phase V-I Measurement3/LConn1 -- Three-Phase Series RLC Branch2/RConn1
  Three-Phase V-I Measurement3/LConn2 -- Three-Phase Series RLC Branch2/RConn2
  Three-Phase V-I Measurement3/LConn3 -- Three-Phase Series RLC Branch2/RConn3
  Three-Phase V-I Measurement4/LConn1 -- Three-Phase Series RLC Branch3/RConn1
  Three-Phase V-I Measurement4/LConn2 -- Three-Phase Series RLC Branch3/RConn2
  Three-Phase V-I Measurement4/LConn3 -- Three-Phase Series RLC Branch3/RConn3
  Three-Phase Breaker/RConn1 -- Three-Phase Series RLC Branch6/LConn1
  Three-Phase Breaker/RConn2 -- Three-Phase Series RLC Branch6/LConn2
  Three-Phase Series RLC Branch6/LConn3 -- Three-Phase Breaker/RConn3
  Three-Phase Breaker/LConn1 -- Three-Phase V-I Measurement1/LConn1
  Three-Phase Breaker/LConn2 -- Three-Phase V-I Measurement1/LConn2
  Three-Phase Breaker/LConn3 -- Three-Phase V-I Measurement1/LConn3
  Three-Phase Series RLC Branch7/RConn1 -- Three-Phase Breaker1/LConn1
  Three-Phase Series RLC Branch7/RConn2 -- Three-Phase Breaker1/LConn2
  Three-Phase Series RLC Branch7/RConn3 -- Three-Phase Breaker1/LConn3
  Three-Phase Breaker1/RConn3 -- Three-Phase V-I Measurement/LConn3
  Three-Phase Breaker1/RConn2 -- Three-Phase V-I Measurement/LConn2
  Three-Phase Breaker1/RConn1 -- Three-Phase V-I Measurement/LConn1
  Breaker4/RConn1 -- Three-Phase Series RLC Branch8/LConn2
  Three-Phase Series RLC Branch8/LConn1 -- Breaker3/RConn1
  Breaker5/RConn1 -- Three-Phase Series RLC Branch8/LConn3
  Ground1/LConn1 -- Three-Phase Series RLC Branch8/RConn1 -- Three-Phase Series RLC Branch8/RConn2 -- Three-Phase Series RLC Branch8/RConn3
  Variant Subsystem3/RConn3 -- Three-Phase Series RLC Branch3/LConn3
  Variant Subsystem3/RConn2 -- Three-Phase Series RLC Branch3/LConn2
  Variant Subsystem3/RConn1 -- Three-Phase Series RLC Branch3/LConn1
  Variant Subsystem2/RConn2 -- Three-Phase Series RLC Branch2/LConn2
  Variant Subsystem2/RConn1 -- Three-Phase Series RLC Branch2/LConn1
  Variant Subsystem2/RConn3 -- Three-Phase Series RLC Branch2/LConn3
  Variant Subsystem1/RConn3 -- Three-Phase Series RLC Branch1/LConn3
  Variant Subsystem1/RConn2 -- Three-Phase Series RLC Branch1/LConn2
  Variant Subsystem1/RConn1 -- Three-Phase Series RLC Branch1/LConn1
  Three-Phase Series RLC Branch7/LConn1 -- Three-Phase V-I Measurement5/RConn1
  Three-Phase V-I Measurement5/RConn2 -- Three-Phase Series RLC Branch7/LConn2
  Three-Phase Series RLC Branch7/LConn3 -- Three-Phase V-I Measurement5/RConn3

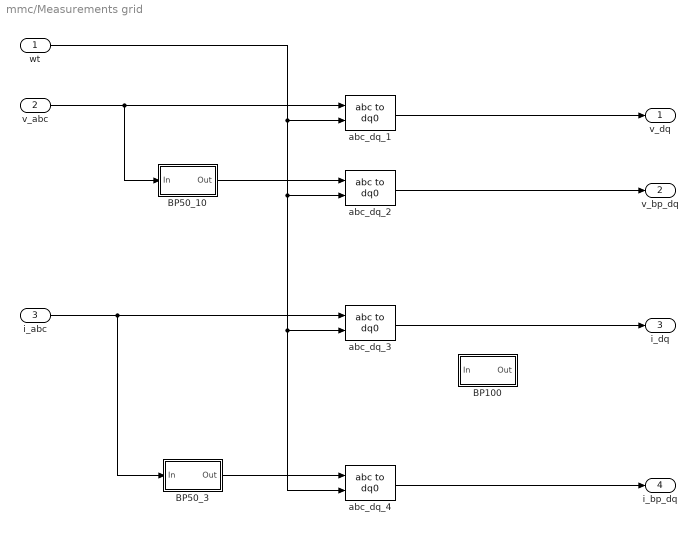
== system mmc/Measurements grid ==
  wt : Inport
  v_abc : Inport  Port=2
  i_abc : Inport  Port=3
  BP100 : Subsystem  DialogController=fdesignblkfcn  InitFcn=fdesignblkfcn(gcbh, {'InitFcn'});  mask(Bandpass Filter){}
      mask help: dsp:DSPFilterDesignBlockDialog:BandpassFdesign_MaskDesc
      settings: CopyFcn=fdesignblkfcn(gcbh, {'CopyFcn'});
      mask Help: helpview(mapfilelocation('dsp'), 'dspbandpassfilter');
      mask Display: disp('Bandpass');
  BP50_10 : Subsystem  DialogController=fdesignblkfcn  InitFcn=fdesignblkfcn(gcbh, {'InitFcn'});  mask(Bandpass Filter){}
      mask help: dsp:DSPFilterDesignBlockDialog:BandpassFdesign_MaskDesc
      settings: CopyFcn=fdesignblkfcn(gcbh, {'CopyFcn'});
      mask Help: helpview(mapfilelocation('dsp'), 'dspbandpassfilter');
      mask Display: disp('Bandpass');
  BP50_3 : Subsystem  DialogController=fdesignblkfcn  InitFcn=fdesignblkfcn(gcbh, {'InitFcn'});  mask(Bandpass Filter){}
      mask help: dsp:DSPFilterDesignBlockDialog:BandpassFdesign_MaskDesc
      settings: CopyFcn=fdesignblkfcn(gcbh, {'CopyFcn'});
      mask Help: helpview(mapfilelocation('dsp'), 'dspbandpassfilter');
      mask Display: disp('Bandpass');
  abc_dq_{1..4} (4 alike) : spsabctodq0Lib/abc to dq0  Alignment=Aligned with phase A axis
  v_dq : Outport
  v_bp_dq : Outport  Port=2
  i_dq : Outport  Port=3
  i_bp_dq : Outport  Port=4
  wires:
  abc_dq_1/1 -> v_dq/1
  v_abc/1 -> BP50_10/1(In), abc_dq_1/1
  abc_dq_4/1 -> i_bp_dq/1
  i_abc/1 -> BP50_3/1(In), abc_dq_3/1
  abc_dq_2/1 -> v_bp_dq/1
  wt/1 -> abc_dq_1/2, abc_dq_3/2, abc_dq_4/2, abc_dq_2/2
  BP50_10/1(Out) -> abc_dq_2/1
  BP50_3/1(Out) -> abc_dq_4/1
  abc_dq_3/1 -> i_dq/1

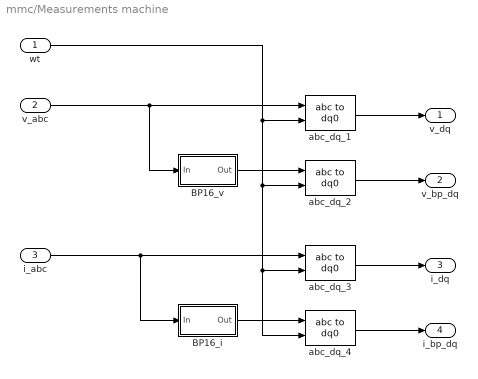
== system mmc/Measurements machine ==
  wt : Inport
  v_abc : Inport  Port=2
  i_abc : Inport  Port=3
  BP16_i : Subsystem  DialogController=fdesignblkfcn  InitFcn=fdesignblkfcn(gcbh, {'InitFcn'});  mask(Bandpass Filter){}
      mask help: dsp:DSPFilterDesignBlockDialog:BandpassFdesign_MaskDesc
      settings: CopyFcn=fdesignblkfcn(gcbh, {'CopyFcn'});
      mask Help: helpview(mapfilelocation('dsp'), 'dspbandpassfilter');
      mask Display: disp('Bandpass');
  BP16_v : Subsystem  DialogController=fdesignblkfcn  InitFcn=fdesignblkfcn(gcbh, {'InitFcn'});  mask(Bandpass Filter){}
      mask help: dsp:DSPFilterDesignBlockDialog:BandpassFdesign_MaskDesc
      settings: CopyFcn=fdesignblkfcn(gcbh, {'CopyFcn'});
      mask Help: helpview(mapfilelocation('dsp'), 'dspbandpassfilter');
      mask Display: disp('Bandpass');
  abc_dq_{1..4} (4 alike) : spsabctodq0Lib/abc to dq0  Alignment=Aligned with phase A axis
  v_dq : Outport
  v_bp_dq : Outport  Port=2
  i_dq : Outport  Port=3
  i_bp_dq : Outport  Port=4
  wires:
  BP16_i/1(Out) -> abc_dq_4/1
  i_abc/1 -> BP16_i/1(In), abc_dq_3/1
  wt/1 -> abc_dq_1/2, abc_dq_3/2, abc_dq_4/2, abc_dq_2/2
  abc_dq_3/1 -> i_dq/1
  abc_dq_1/1 -> v_dq/1
  abc_dq_4/1 -> i_bp_dq/1
  abc_dq_2/1 -> v_bp_dq/1
  BP16_v/1(Out) -> abc_dq_2/1
  v_abc/1 -> abc_dq_1/1, BP16_v/1(In)

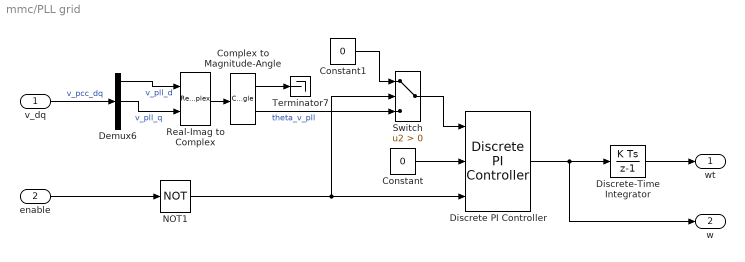
== system mmc/PLL grid ==
  v_dq : Inport
  enable : Inport  Port=2
  Complex to Magnitude-Angle : ComplexToMagnitudeAngle
  Constant : Constant  Value=0
  Constant1 : Constant  Value=0
  Demux6 : Demux  Outputs=3
  Discrete PI Controller : eeDiscretePi/Discrete PI Controller  Kp=ctrl.grid.pll.kp  Ki=ctrl.grid.pll.ki  Kaw=1  x0=ctrl.grid.pll.init_w  Ts=-1
      settings: LibrarySourceBlock=ee_sl_lib/General Control/Discrete PI Controller
  Discrete-Time Integrator : DiscreteIntegrator  gainval=grid.w  SampleTime=-1  ICPrevOutput=DiscIntNeverNeededParam  ICPrevScaledInput=DiscIntNeverNeededParam
  NOT1 : Logic  Operator=NOT  IconShape=distinctive  AllPortsSameDT=off  OutDataTypeStr=boolean
  Real-Imag to Complex : RealImagToComplex
  Switch : Switch  Criteria=u2 > Threshold  SaturateOnIntegerOverflow=off  InputSameDT=off
  Terminator7 : Terminator
  wt : Outport
  w : Outport  Port=2
  wires:
  v_dq/1 -> Demux6/1  "v_pcc_dq"
  Complex to Magnitude-Angle/1 -> Terminator7/1
  Demux6/2 -> Real-Imag to Complex/2  "v_pll_q"
  Complex to Magnitude-Angle/2 -> Switch/3  "theta_v_pll"
  Real-Imag to Complex/1 -> Complex to Magnitude-Angle/1
  Demux6/1 -> Real-Imag to Complex/1  "v_pll_d"
  Constant/1 -> Discrete PI Controller/2
  Discrete PI Controller/1 -> w/1, Discrete-Time Integrator/1
  Discrete-Time Integrator/1 -> wt/1
  NOT1/1 -> Switch/2, Discrete PI Controller/3
  enable/1 -> NOT1/1
  Switch/1 -> Discrete PI Controller/1
  Constant1/1 -> Switch/1

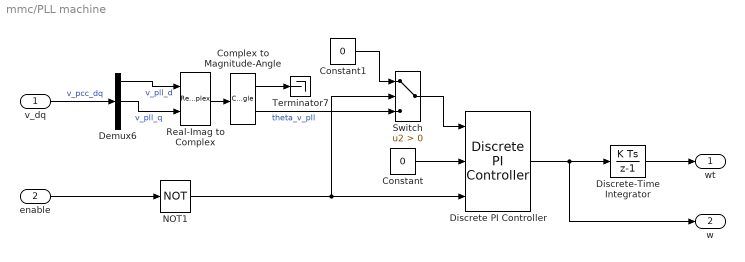
== system mmc/PLL machine ==
  v_dq : Inport
  enable : Inport  Port=2
  Complex to Magnitude-Angle : ComplexToMagnitudeAngle
  Constant : Constant  Value=0
  Constant1 : Constant  Value=0
  Demux6 : Demux  Outputs=3
  Discrete PI Controller : eeDiscretePi/Discrete PI Controller  Kp=ctrl.machine.pll.kp  Ki=ctrl.machine.pll.ki  Kaw=1  x0=ctrl.machine.pll.init_w  Ts=-1
      settings: LibrarySourceBlock=ee_sl_lib/General Control/Discrete PI Controller
  Discrete-Time Integrator : DiscreteIntegrator  gainval=machine.w  SampleTime=-1  ICPrevOutput=DiscIntNeverNeededParam  ICPrevScaledInput=DiscIntNeverNeededParam
  NOT1 : Logic  Operator=NOT  IconShape=distinctive  AllPortsSameDT=off  OutDataTypeStr=boolean
  Real-Imag to Complex : RealImagToComplex
  Switch : Switch  Criteria=u2 > Threshold  SaturateOnIntegerOverflow=off  InputSameDT=off
  Terminator7 : Terminator
  wt : Outport
  w : Outport  Port=2
  wires:
  v_dq/1 -> Demux6/1  "v_pcc_dq"
  Complex to Magnitude-Angle/1 -> Terminator7/1
  Demux6/2 -> Real-Imag to Complex/2  "v_pll_q"
  Complex to Magnitude-Angle/2 -> Switch/3  "theta_v_pll"
  Real-Imag to Complex/1 -> Complex to Magnitude-Angle/1
  Demux6/1 -> Real-Imag to Complex/1  "v_pll_d"
  Constant/1 -> Discrete PI Controller/2
  Discrete PI Controller/1 -> w/1, Discrete-Time Integrator/1
  Discrete-Time Integrator/1 -> wt/1
  NOT1/1 -> Switch/2, Discrete PI Controller/3
  enable/1 -> NOT1/1
  Switch/1 -> Discrete PI Controller/1
  Constant1/1 -> Switch/1

== system mmc/circulating current controller3 ==
  u_ref : Inport
  u : Inport  Port=2
  antiwind : Inport  Port=3
  enable : Inport  Port=4
  Constant1 : Constant  Value=[0 0 0 0]
  NOT1 : Logic  Operator=NOT  IconShape=distinctive  AllPortsSameDT=off  OutDataTypeStr=boolean
  PICtrl : eeDiscretePi/Discrete PI Controller  Kp=ctrl.grid.ictrl.kp  Ki=ctrl.grid.ictrl.ki*0  Kaw=100  x0=0  Ts=-1
      settings: LibrarySourceBlock=ee_sl_lib/General Control/Discrete PI Controller
  Sum : Sum  Inputs=|+-
  Switch : Switch  Criteria=u2 > Threshold  SaturateOnIntegerOverflow=off  InputSameDT=off
  y : Outport
  wires:
  u_ref/1 -> Sum/1
  u/1 -> Sum/2
  NOT1/1 -> Switch/2, PICtrl/3
  enable/1 -> NOT1/1
  PICtrl/1 -> y/1  "y"
  antiwind/1 -> PICtrl/2
  Sum/1 -> Switch/3
  Constant1/1 -> Switch/1
  Switch/1 -> PICtrl/1

== system mmc/dq_to_ab_g ==
  in : Inport
  wt : Inport  Port=2
  Demux1 : Demux  Outputs=2
  Demux16 : Demux  Outputs=2
  Mux11 : Mux
  Selector : Selector  InputPortWidth=4  IndexOptions=Index vector (dialog)  Indices=[1 3]  OutputSizes=1
  Selector1 : Selector  InputPortWidth=4  IndexOptions=Index vector (dialog)  Indices=[2 4]  OutputSizes=1
  Subsystem : Subsystem
  Subsystem1 : Subsystem
  out : Outport
  wires:
  Selector/1 -> Subsystem/1(dq)
  Demux16/2 -> Mux11/3
  in/1 -> Selector1/1, Selector/1
  Subsystem/1(alpha_beta) -> Demux16/1
  Demux16/1 -> Mux11/1
  Mux11/1 -> out/1
  wt/1 -> Subsystem1/2(wt), Subsystem/2(wt)
  Selector1/1 -> Subsystem1/1(dq)
  Subsystem1/1(alpha_beta) -> Demux1/1
  Demux1/1 -> Mux11/2
  Demux1/2 -> Mux11/4

== system mmc/dq_to_ab_m ==
  in : Inport
  wt : Inport  Port=2
  Demux1 : Demux  Outputs=2
  Demux16 : Demux  Outputs=2
  Mux11 : Mux
  Selector : Selector  InputPortWidth=4  IndexOptions=Index vector (dialog)  Indices=[1 3]  OutputSizes=1
  Selector1 : Selector  InputPortWidth=4  IndexOptions=Index vector (dialog)  Indices=[2 4]  OutputSizes=1
  Subsystem : Subsystem
  Subsystem1 : Subsystem
  out : Outport
  wires:
  Selector/1 -> Subsystem/1(dq)
  Demux16/2 -> Mux11/3
  in/1 -> Selector1/1, Selector/1
  Subsystem/1(alpha_beta) -> Demux16/1
  Demux16/1 -> Mux11/1
  Mux11/1 -> out/1
  wt/1 -> Subsystem1/2(wt), Subsystem/2(wt)
  Selector1/1 -> Subsystem1/1(dq)
  Subsystem1/1(alpha_beta) -> Demux1/1
  Demux1/1 -> Mux11/2
  Demux1/2 -> Mux11/4

== system mmc/dq_to_ab_ns ==
  in : Inport
  wt : Inport  Port=2
  Demux1 : Demux  Outputs=2
  Demux16 : Demux  Outputs=2
  Mux11 : Mux
  Selector : Selector  InputPortWidth=4  IndexOptions=Index vector (dialog)  Indices=[1 3]  OutputSizes=1
  Selector1 : Selector  InputPortWidth=4  IndexOptions=Index vector (dialog)  Indices=[2 4]  OutputSizes=1
  Subsystem : Subsystem
  Subsystem1 : Subsystem
  out : Outport
  wires:
  Selector/1 -> Subsystem/1(dq)
  Demux16/2 -> Mux11/3
  in/1 -> Selector1/1, Selector/1
  Subsystem/1(alpha_beta) -> Demux16/1
  Demux16/1 -> Mux11/1
  Mux11/1 -> out/1
  wt/1 -> Subsystem1/2(wt), Subsystem/2(wt)
  Selector1/1 -> Subsystem1/1(dq)
  Subsystem1/1(alpha_beta) -> Demux1/1
  Demux1/1 -> Mux11/2
  Demux1/2 -> Mux11/4

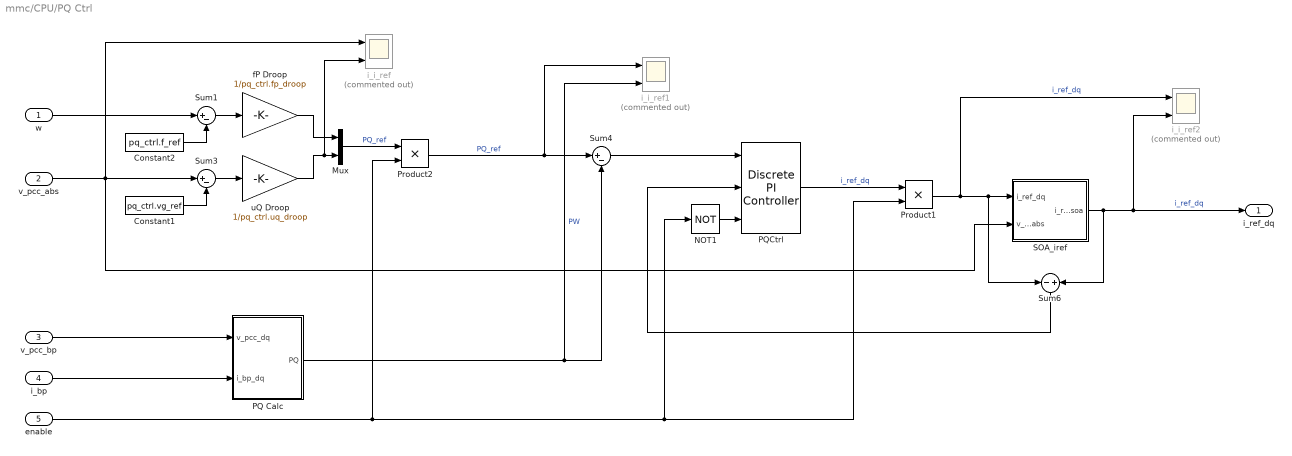
== system mmc/CPU/PQ Ctrl ==
  w : Inport
  v_pcc_abs : Inport  Port=2
  v_pcc_bp : Inport  Port=3
  i_bp : Inport  Port=4
  enable : Inport  Port=5
  Constant1 : Constant  Value=pq_ctrl.vg_ref
  Constant2 : Constant  Value=pq_ctrl.f_ref
  Mux : Mux  Inputs=2
  NOT1 : Logic  Operator=NOT  IconShape=distinctive  AllPortsSameDT=off  OutDataTypeStr=boolean
  PQ Calc : Subsystem
  PQCtrl : eeDiscretePi/Discrete PI Controller  Kp=pq_ctrl.kp  Ki=pq_ctrl.ki  Kaw=100  x0=0  Ts=-1
      settings: LibrarySourceBlock=ee_sl_lib/General Control/Discrete PI Controller
  Product1 : Product
  Product2 : Product
  SOA_iref : Subsystem
  Sum1 : Sum  Inputs=|+-
  Sum3 : Sum  Inputs=|+-
  Sum4 : Sum  Inputs=|+-
  Sum6 : Sum  Inputs=-|+
  fP Droop : Gain  Gain=1/pq_ctrl.fp_droop
  i_i_ref : Scope  Commented=on  NumInputPorts=2
  i_i_ref1 : Scope  Commented=on  NumInputPorts=2
  i_i_ref2 : Scope  Commented=on  NumInputPorts=2
  uQ Droop : Gain  Gain=1/pq_ctrl.uq_droop
  i_ref_dq : Outport
  wires:
  Sum6/1 -> PQCtrl/2
  Product1/1 -> i_i_ref2/1, SOA_iref/1(i_ref_dq), Sum6/1  "i_ref_dq"
  fP Droop/1 -> Mux/1
  SOA_iref/1(i_ref_dq_soa) -> i_i_ref2/2, i_ref_dq/1, Sum6/2  "i_ref_dq"
  uQ Droop/1 -> i_i_ref/2, Mux/2
  Sum3/1 -> uQ Droop/1
  enable/1 -> NOT1/1, Product1/2, Product2/2
  PQCtrl/1 -> Product1/1  "i_ref_dq"
  Mux/1 -> Product2/1  "PQ_ref"
  v_pcc_abs/1 -> i_i_ref/1, SOA_iref/2(v_pcc_abs), Sum3/1
  Product2/1 -> i_i_ref1/1, Sum4/1  "PQ_ref"
  PQ Calc/1(PQ) -> i_i_ref1/2, Sum4/2  "PW"
  Constant2/1 -> Sum1/2
  Sum1/1 -> fP Droop/1
  Sum4/1 -> PQCtrl/1
  Constant1/1 -> Sum3/2
  NOT1/1 -> PQCtrl/3
  v_pcc_bp/1 -> PQ Calc/1(v_pcc_dq)
  w/1 -> Sum1/1
  i_bp/1 -> PQ Calc/2(i_bp_dq)

== system mmc/CPU/Subsystem ==
  x : Inport
  y : Inport  Port=2
  Demux : Demux  Outputs=2
  Demux1 : Demux  Outputs=2
  Mux1 : Mux  Inputs=2
  Mux2 : Mux  Inputs=2
  d : Outport
  q : Outport  Port=2
  wires:
  Mux2/1 -> q/1
  y/1 -> Demux1/1
  Demux/2 -> Mux2/1
  Demux1/2 -> Mux2/2
  Demux/1 -> Mux1/1
  Demux1/1 -> Mux1/2
  Mux1/1 -> d/1
  x/1 -> Demux/1

== system mmc/CPU/Subsystem1 ==
  x : Inport
  y : Inport  Port=2
  Demux : Demux  Outputs=2
  Demux1 : Demux  Outputs=2
  Mux1 : Mux  Inputs=2
  Mux2 : Mux  Inputs=2
  d : Outport
  q : Outport  Port=2
  wires:
  Mux2/1 -> q/1
  y/1 -> Demux1/1
  Demux/2 -> Mux2/1
  Demux1/2 -> Mux2/2
  Demux/1 -> Mux1/1
  Demux1/1 -> Mux1/2
  Mux1/1 -> d/1
  x/1 -> Demux/1

== system mmc/CPU/Subsystem2 ==
  i_dq : Inport
  w : Inport  Port=2
  Gain : Gain  Gain=J  Multiplication=Matrix(K*u) (u vector)
  Gain1 : Gain  Gain=grid.tr.l
  Gain2 : Gain  Gain=grid.tr.r
  Product : Product
  Sum8 : Sum  Inputs=++|
  dm_dq : Outport
  wires:
  Gain1/1 -> Sum8/2
  Sum8/1 -> dm_dq/1  "dm_dq"
  Product/1 -> Gain/1
  Gain/1 -> Gain1/1  "dm_dq"
  w/1 -> Product/1
  i_dq/1 -> Gain2/1, Product/2
  Gain2/1 -> Sum8/1

== system mmc/CPU/Subsystem3 ==
  i_dq : Inport
  w : Inport  Port=2
  Gain : Gain  Gain=J  Multiplication=Matrix(K*u) (u vector)
  Gain1 : Gain  Gain=machine.tr.l
  Gain2 : Gain  Gain=machine.tr.r
  Product : Product
  Sum8 : Sum  Inputs=++|
  dm_dq : Outport
  wires:
  Gain1/1 -> Sum8/2
  Sum8/1 -> dm_dq/1  "dm_dq"
  Product/1 -> Gain/1
  Gain/1 -> Gain1/1  "dm_dq"
  w/1 -> Product/1
  i_dq/1 -> Gain2/1, Product/2
  Gain2/1 -> Sum8/1

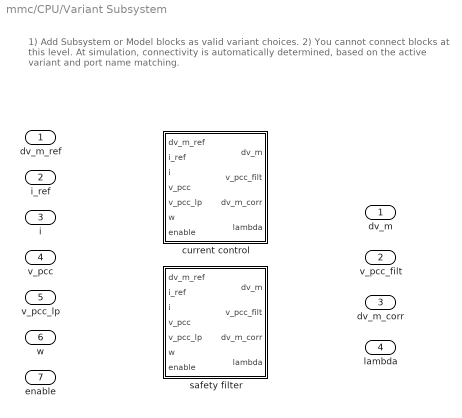
== system mmc/CPU/Variant Subsystem ==
  note: 1) Add Subsystem or Model blocks as valid variant choices.
      | 2) You cannot connect blocks at this level. At simulation, connectivity is automatically
      | determined, based on the active variant and port name matching.
  dv_m_ref : Inport
  i_ref : Inport  Port=2
  i : Inport  Port=3
  v_pcc : Inport  Port=4
  v_pcc_lp : Inport  Port=5
  w : Inport  Port=6
  enable : Inport  Port=7
  current control : Subsystem  VariantControl=ctrl.machine.ictrl.sel==0
  safety filter : Subsystem  VariantControl=ctrl.machine.ictrl.sel==1
  dv_m : Outport
  v_pcc_filt : Outport  Port=2
  dv_m_corr : Outport  Port=3
  lambda : Outport  Port=4

== system mmc/CPU/ab_to_ab0 ==
  In1 : Inport
  Constant8 : Constant  Value=0
  Demux : Demux  Outputs=2
  Mux7 : Mux  Inputs=3
  Out1 : Outport
  wires:
  Demux/1 -> Mux7/1
  Demux/2 -> Mux7/2
  Constant8/1 -> Mux7/3
  In1/1 -> Demux/1
  Mux7/1 -> Out1/1

== system mmc/CPU/ab_to_ab1 ==
  In1 : Inport
  Constant8 : Constant  Value=0
  Demux : Demux  Outputs=2
  Mux7 : Mux  Inputs=3
  Out1 : Outport
  wires:
  Demux/1 -> Mux7/1
  Demux/2 -> Mux7/2
  Constant8/1 -> Mux7/3
  In1/1 -> Demux/1
  Mux7/1 -> Out1/1

== system mmc/CPU/ab_to_ab2 ==
  i_ref_dq : Inport
  Constant8 : Constant  Value=0
  Demux : Demux  Outputs=2
  Mux7 : Mux  Inputs=3
  Out1 : Outport
  wires:
  Demux/1 -> Mux7/1
  Demux/2 -> Mux7/2
  Constant8/1 -> Mux7/3
  i_ref_dq/1 -> Demux/1
  Mux7/1 -> Out1/1
